simulink model "CRITIS_1_full"  (R2022b)
settings: Solver=VariableStepAuto  StartTime=0.0  StopTime=7  RelTol=1e-3
(part 13 of 13)

== matlab function CRITIS_1_full/TELCOMMUNICATIONS2/Subsystem5/MATLAB Function2 ==
  data: se output double size=1; se_vect output; servizio input; consumed input; operation1 input; operation2 input; num_serv input; out_service input
function [se,se_vect] = Dep(servizio,consumed,operation1,operation2,num_serv,out_service)

Service_Fault=zeros(1,5);

for i=1:num_serv

    if operation1==1 % AND
        
        Service_Fault(i)=max(abs(consumed(i,:).*servizio(i,:)-consumed(i,:)));
    else % OR
        
        Service_Fault(i)=1-max(abs(consumed(i,:).*servizio(i,:)));
    end
    
end


se=1-Service_Fault(1);

if num_serv>1
    for i=2:num_serv

      if operation2==1 % AND
        se=min(se,1-Service_Fault(i));
      else % OR
        se=max(se,1-Service_Fault(i));
      end

    end
end

se_vect=zeros(1,20);
if out_service>1
    se_vect(out_service-1)=se;
end

== matlab function CRITIS_1_full/TELCOMMUNICATIONS1/Subsystem6/MATLAB Function2 ==
  data: se output double size=1; se_vect output; servizio input; consumed input; operation1 input; operation2 input; num_serv input; out_service input; Service_Fault output
function [se,se_vect,Service_Fault] = Dep(servizio,consumed,operation1,operation2,num_serv,out_service)

Service_Fault=zeros(1,5);

for i=1:num_serv

    if operation1==1 % AND
        
        Service_Fault(i)=max(abs(consumed(:,i).*servizio(:,i)-consumed(:,i)));
      
    else % OR
        
        Service_Fault(i)=1-max(abs(consumed(:,i).*servizio(:,i)));
    end
    
end


se=1-Service_Fault(1);

if num_serv>1
    for i=2:num_serv

      if operation2==1 % AND
        se=min(se,1-Service_Fault(i));
      else % OR
        se=max(se,1-Service_Fault(i));
      end

    end
end

se_vect=zeros(1,20);
if out_service>1
    se_vect(out_service-1)=se;
end

== matlab function CRITIS_1_full/ENERGY PROVIDER 1/Subsystem1/MATLAB Function2 ==
  data: se output double size=1; se_vect output; servizio input; consumed input; operation1 input; operation2 input; num_serv input; out_service input; Service_Fault output
function [se,se_vect,Service_Fault] = Dep(servizio,consumed,operation1,operation2,num_serv,out_service)

Service_Fault=zeros(1,5);

for i=1:num_serv

    if operation1==1 % AND
        
        Service_Fault(i)=max(abs(consumed(:,i).*servizio(:,i)-consumed(:,i)));
      
    else % OR
        
        Service_Fault(i)=1-max(abs(consumed(:,i).*servizio(:,i)));
    end
    
end


se=1-Service_Fault(1);

if num_serv>1
    for i=2:num_serv

      if operation2==1 % AND
        se=min(se,1-Service_Fault(i));
      else % OR
        se=max(se,1-Service_Fault(i));
      end

    end
end

se_vect=zeros(1,20);
if out_service>1
    se_vect(out_service-1)=se;
end

== matlab function CRITIS_1_full/BANK 1/maxmin1 ==
  data: u1 input; y output; u2 input
function y = maxmin(u1,u2)

y=[0 0];
y(1) = max(u1(1),u2(1));
y(2) = min(u1(2),u2(2));

== matlab function CRITIS_1_full/DEPARTMENT OF INDUSTRIAL DEVELOPMENT/MISE_Physical ==
  data: N1 input; Physical output
function Physical = f(N1)

Physical = min([N1]);

== matlab function CRITIS_1_full/RAILWAYS/maxmin3 ==
  data: u1 input; y output; u2 input
function y = maxmin(u1,u2)

y=[0 0];
y(1) = max(u1(1),u2(1));
y(2) = min(u1(2),u2(2));

== matlab function CRITIS_1_full/AIR TRANSPORTATION/maxmin1 ==
  data: u1 input; y output; u2 input
function y = maxmin(u1,u2)

y=[0 0];
y(1) = max(u1(1),u2(1));
y(2) = min(u1(2),u2(2));

== matlab function CRITIS_1_full/mean 5 ==
  data: u input; y output
function y = fcn(u)

y=[0 0];
n=length(u)/2;
y(1) = sum(u(1:2:end))/n;
y(2) = sum(u(2:2:end))/n;

== matlab function CRITIS_1_full/AIR TRANSPORTATION/maxmin ==
  data: u1 input; y output; u2 input
function y = maxmin(u1,u2)

y=[0 0];
y(1) = max(u1(1),u2(1));
y(2) = min(u1(2),u2(2));

== matlab function CRITIS_1_full/ENERGY PROVIDER 1/maxmin ==
  data: u1 input; y output; u2 input
function y = maxmin(u1,u2)

y=[0 0];
y(1) = max(u1(1),u2(1));
y(2) = min(u1(2),u2(2));

== matlab function CRITIS_1_full/ENERGY PROVIDER 1/maxmin1 ==
  data: u1 input; y output; u2 input; u3 input
function y = maxmin(u1,u2,u3)

y=[0 0];
y(1) = max([u1(1),u2(1),u3(1)]);
y(2) = min([u1(2),u2(2),u3(2)]);

== matlab function CRITIS_1_full/TELCOMMUNICATIONS1/maxmin ==
  data: u1 input; y output; u2 input
function y = maxmin(u1,u2)

y=[0 0];
y(1) = max(u1(1),u2(1));
y(2) = min(u1(2),u2(2));

== matlab function CRITIS_1_full/TELCOMMUNICATIONS1/maxmin1 ==
  data: u1 input; y output; u2 input
function y = maxmin(u1,u2)

y=[0 0];
y(1) = max(u1(1),u2(1));
y(2) = min(u1(2),u2(2));

== matlab function CRITIS_1_full/RAILWAYS/maxmin ==
  data: u1 input; y output; u2 input
function y = maxmin(u1,u2)

y=[0 0];
y(1) = max(u1(1),u2(1));
y(2) = min(u1(2),u2(2));

== matlab function CRITIS_1_full/TELCOMMUNICATIONS1/TIM_Routing_Switching ==
  data: N1 input; Routing output; N2 input; N3 input; N4 input; N5 input; N6 input; N7 input
function Routing = f(N1,N2,N3,N4,N5,N6,N7)

persistent first_run;

if isempty(first_run)
    first_run=0;
    Routing=1;
else

    Routing=0;

    Routing = min([N1 N2 N3 N4 N5 N6 N7]);

end

== matlab function CRITIS_1_full/RAILWAYS/maxmin1 ==
  data: u1 input; y output; u2 input
function y = maxmin(u1,u2)

y=[0 0];
y(1) = max(u1(1),u2(1));
y(2) = min(u1(2),u2(2));

== matlab function CRITIS_1_full/RAILWAYS/maxmin2 ==
  data: u1 input; y output; u2 input
function y = maxmin(u1,u2)

y=[0 0];
y(1) = max(u1(1),u2(1));
y(2) = min(u1(2),u2(2));

== matlab function CRITIS_1_full/ENERGY PROVIDER 2/maxmin1 ==
  data: u1 input; y output; u2 input; u3 input
function y = maxmin(u1,u2,u3)

y=[0 0];
y(1) = max([u1(1),u2(1),u3(1)]);
y(2) = min([u1(2),u2(2),u3(2)]);

== matlab function CRITIS_1_full/ENERGY PROVIDER 2/maxmin2 ==
  data: u1 input; y output; u2 input
function y = maxmin(u1,u2)

y=[0 0];
y(1) = max(u1(1),u2(1));
y(2) = min(u1(2),u2(2));

== matlab function CRITIS_1_full/DEPARTMENT OF INDUSTRIAL DEVELOPMENT/maxmin1 ==
  data: u1 input; y output; u2 input
function y = maxmin(u1,u2)

y=[0 0];
y(1) = max(u1(1),u2(1));
y(2) = min(u1(2),u2(2));

== matlab function CRITIS_1_full/TELCOMMUNICATIONS2/maxmin1 ==
  data: u1 input; y output; u2 input
function y = maxmin(u1,u2)

y=[0 0];
y(1) = max(u1(1),u2(1));
y(2) = min(u1(2),u2(2));

== matlab function CRITIS_1_full/TELCOMMUNICATIONS2/maxmin2 ==
  data: u1 input; y output; u2 input
function y = maxmin(u1,u2)

y=[0 0];
y(1) = max(u1(1),u2(1));
y(2) = min(u1(2),u2(2));
